simulink model "slb_WFA"  (R2015b)
settings: Solver=FixedStepDiscrete  SolverMode=SingleTasking  StartTime=0.0  StopTime=10.0  RelTol=1e-3
libraries: simulink x1
settings Model: Creator=at-mt  LastModifiedBy=amatsumo
settings DataIOCC: SaveFormat=Array  SignalLoggingSaveFormat=ModelDataLogs  SaveOutput=off  SignalLogging=off  SaveTime=off
settings OptimizationCC: BlockReduction=off  ConditionallyExecuteInputs=off  DefaultParameterBehavior=Inlined  ExpressionDepthLimit=2147483647
settings DebuggingCC: AlgebraicLoopMsg=error  UnderspecifiedInitializationDetection=Classic  MergeDetectMultiDrivingBlocksExec=none  SolverPrmCheckMsg=warning  MultiTaskDSMMsg=warning  MultiTaskCondExecSysMsg=none  SingleTaskRateTransMsg=error  ParameterOverflowMsg=warning  FcnCallInpInsideContextMsg=EnableAllAsWarning  StateNameClashWarn=warning
settings HardwareCC: ProdBitPerPointer=32  ProdLargestAtomicFloat=None  ProdIntDivRoundTo=Undefined  ProdEndianess=Unspecified  ProdWordSize=32  ProdHWDeviceType=ASIC/FPGA->ASIC/FPGA  ProdEqTarget=off
settings GRTTargetCC: GeneratePreprocessorConditionals=Disable all  CombineOutputUpdateFcns=off  GRTInterface=on
settings ConfigComp: CovModelRefEnable=Off  CovSFcnEnable=off

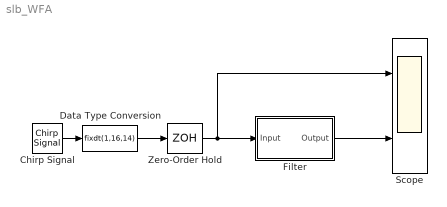
== system slb_WFA ==
  Chirp Signal : simulink/Sources/Chirp Signal  f1=10  T=10  f2=500
  Data Type Conversion : DataTypeConversion  OutDataTypeStr=fixdt(1,16,14)  RndMeth=Nearest
  Filter : Subsystem  Tag=FilterWizardSubSystem
      settings: ErrorFcn=dspFilterRealizedInBasicElemsAlgLoopErrFcnCallback
  Scope : Scope  NumInputPorts=2
  Zero-Order Hold : ZeroOrderHold  SampleTime=1/1000
  wires:
  Chirp Signal/1 -> Data Type Conversion/1
  Zero-Order Hold/1 -> Scope/1, Filter/1(Input)
  Data Type Conversion/1 -> Zero-Order Hold/1
  Filter/1(Output) -> Scope/2

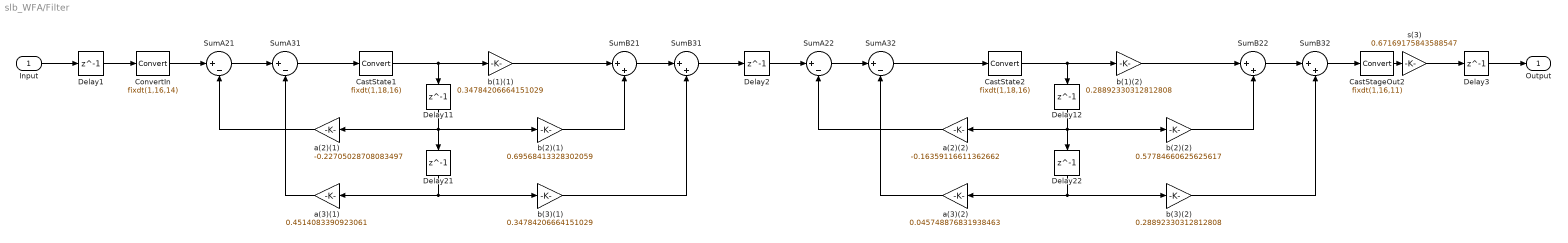
== system slb_WFA/Filter ==
  Input : Inport
  CastStageOut2 : DataTypeConversion  OutDataTypeStr=fixdt(1,16,11)  RndMeth=Nearest
  CastState1 : DataTypeConversion  OutDataTypeStr=fixdt(1,18,16)  RndMeth=Nearest
  CastState2 : DataTypeConversion  OutDataTypeStr=fixdt(1,18,16)  RndMeth=Nearest
  ConvertIn : DataTypeConversion  OutDataTypeStr=fixdt(1,16,14)  RndMeth=Nearest  SaturateOnIntegerOverflow=on
  Delay{1..3,11..12,21..22} (7 alike) : Delay  DelayLength=1  InitialCondition=0
  SumA{21..22,31..32} (4 alike) : Sum  Inputs=|+-  AccumDataTypeStr=fixdt(1,36,30)  OutDataTypeStr=fixdt(1,36,30)  RndMeth=Nearest
  SumB{21..22,31..32} (4 alike) : Sum  Inputs=|++  AccumDataTypeStr=fixdt(1,36,31)  OutDataTypeStr=fixdt(1,36,31)  RndMeth=Nearest
  a(2)(1) : Gain  Gain=-0.22705028708083497  ParamDataTypeStr=fixdt(1,16,14)  OutDataTypeStr=fixdt(1,34,30)  RndMeth=Nearest
  a(2)(2) : Gain  Gain=-0.16359116611362662  ParamDataTypeStr=fixdt(1,16,14)  OutDataTypeStr=fixdt(1,34,30)  RndMeth=Nearest
  a(3)(1) : Gain  Gain=0.4514083390923061  ParamDataTypeStr=fixdt(1,16,14)  OutDataTypeStr=fixdt(1,34,30)  RndMeth=Nearest
  a(3)(2) : Gain  Gain=0.045748876831938463  ParamDataTypeStr=fixdt(1,16,14)  OutDataTypeStr=fixdt(1,34,30)  RndMeth=Nearest
  b(1)(1) : Gain  Gain=0.34784206664151029  ParamDataTypeStr=fixdt(1,16,15)  OutDataTypeStr=fixdt(1,34,31)  RndMeth=Nearest
  b(1)(2) : Gain  Gain=0.28892330312812808  ParamDataTypeStr=fixdt(1,16,15)  OutDataTypeStr=fixdt(1,34,31)  RndMeth=Nearest
  b(2)(1) : Gain  Gain=0.69568413328302059  ParamDataTypeStr=fixdt(1,16,15)  OutDataTypeStr=fixdt(1,34,31)  RndMeth=Nearest
  b(2)(2) : Gain  Gain=0.57784660625625617  ParamDataTypeStr=fixdt(1,16,15)  OutDataTypeStr=fixdt(1,34,31)  RndMeth=Nearest
  b(3)(1) : Gain  Gain=0.34784206664151029  ParamDataTypeStr=fixdt(1,16,15)  OutDataTypeStr=fixdt(1,34,31)  RndMeth=Nearest
  b(3)(2) : Gain  Gain=0.28892330312812808  ParamDataTypeStr=fixdt(1,16,15)  OutDataTypeStr=fixdt(1,34,31)  RndMeth=Nearest
  s(3) : Gain  Gain=0.67169175843588547  ParamDataTypeStr=fixdt(1,16,15)  OutDataTypeStr=fixdt(1,18,13)  RndMeth=Nearest
  Output : Outport
  wires:
  Delay3/1 -> Output/1
  Delay1/1 -> ConvertIn/1
  CastStageOut2/1 -> s(3)/1
  s(3)/1 -> Delay3/1
  b(3)(2)/1 -> SumB32/2
  Delay22/1 -> b(3)(2)/1, a(3)(2)/1
  a(3)(2)/1 -> SumA32/2
  b(2)(2)/1 -> SumB22/2
  Delay12/1 -> Delay22/1, b(2)(2)/1, a(2)(2)/1
  a(2)(2)/1 -> SumA22/2
  SumB32/1 -> CastStageOut2/1
  SumB22/1 -> SumB32/1
  b(1)(2)/1 -> SumB22/1
  CastState2/1 -> Delay12/1, b(1)(2)/1
  SumA32/1 -> CastState2/1
  SumA22/1 -> SumA32/1
  Delay2/1 -> SumA22/1
  ConvertIn/1 -> SumA21/1
  b(3)(1)/1 -> SumB31/2
  Delay21/1 -> b(3)(1)/1, a(3)(1)/1
  a(3)(1)/1 -> SumA31/2
  b(2)(1)/1 -> SumB21/2
  Delay11/1 -> Delay21/1, b(2)(1)/1, a(2)(1)/1
  a(2)(1)/1 -> SumA21/2
  SumB31/1 -> Delay2/1
  SumB21/1 -> SumB31/1
  b(1)(1)/1 -> SumB21/1
  CastState1/1 -> Delay11/1, b(1)(1)/1
  SumA31/1 -> CastState1/1
  SumA21/1 -> SumA31/1
  Input/1 -> Delay1/1
